simulink model "foc_control"  (R2022b)
settings: Solver=FixedStepAuto  StartTime=0.0  StopTime=0.1  FixedStep=1e-6  RelTol=1e-3
InitFcn:
  | init_pmsm
values from neighbouring files (symbols this model uses):
  B = 0.00001    (= 1e-05)    [init_pmsm.m]
  current_loop_wc = 800    [init_pmsm.m]
  J = 0.0001    [init_pmsm.m]
  Ld = 0.0028    [init_pmsm.m]
  Lq = 0.0028    [init_pmsm.m]
  Pn = 7    [init_pmsm.m]
  Psi = 0.002188    [init_pmsm.m]
  Rs = 5.1    [init_pmsm.m]
  Ts = 1/PWM_Freq    (= 0.000125)    [init_pmsm.m]
  Udc = 12    [init_pmsm.m]
libraries: slpidlib x2, mcbcontrolslib x1, simulink x1
settings Model: Creator=w1545  LastModifiedBy=w1545

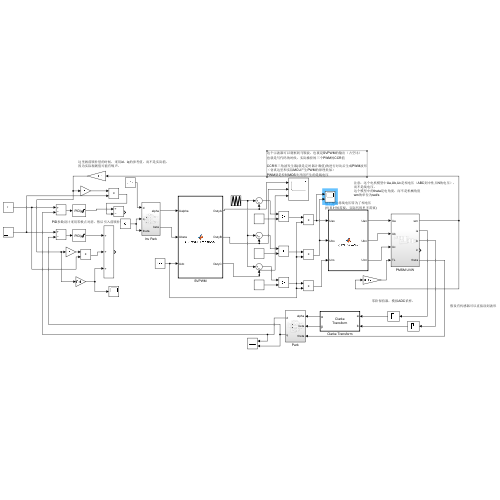
[thumbnail: Simulink's stored preview of the top-level diagram]
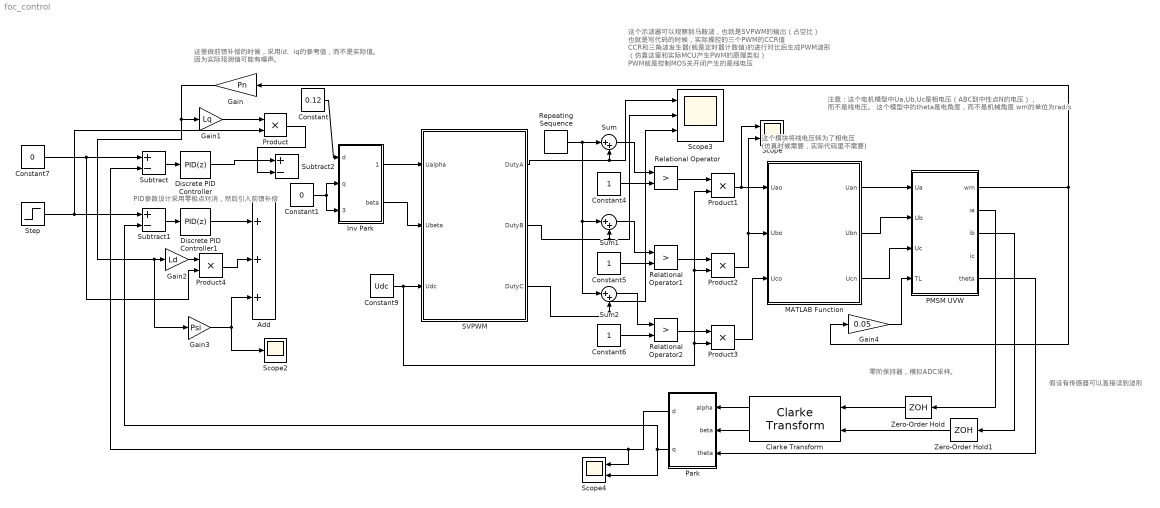
== system foc_control ==
  note: PID参数设计采用零极点对消，然后引入前馈补偿
  note: 假设有传感器可以直接读到波形
  note: 零阶保持器，模拟ADC采样。
  note: 这个模块将线电压转为了相电压
      | (仿真时候需要，实际代码里不需要)
  note: 这个示波器可以观察到马鞍波，也就是SVPWM的输出（占空比）
      | 也就是写代码的时候，实际操控的三个PWM的CCR值
      |
      | CCR和三角波发生器(就是定时器计数值)的进行对比后生成PWM波形
      | （仿真这里和实际MCU产生PWM的原理类似）
      | PWM就是控制MOS关开闭产生的是线电压
  note: 这里做前馈补偿的时候，采用id、iq的参考值，而不是实际值。
      | 因为实际观测值可能有噪声。
  note: 注意：这个电机模型中Ua,Ub,Uc是相电压（ABC到中性点N的电压），
      | 而不是线电压。
      | 这个模型中的theta是电角度，而不是机械角度
      | wm的单位为rad/s
  Add : Sum  Inputs=+++
  Clarke Transform : mcbcontrolslib/Clarke Transform  VariantControl=Variant2
      settings: LibrarySourceBlock=mcbhdllib/Controls/Math Transforms/Clarke Transform
  Constant : Constant  Value=0.12
  Constant1 : Constant  Value=0
  Constant4 : Constant
  Constant5 : Constant
  Constant6 : Constant
  Constant7 : Constant  Value=0
  Constant9 : Constant  Value=Udc
  Discrete PID Controller : slpidlib/PID Controller  Controller=PID  Form=Parallel  TimeDomain=Discrete-time  UseExternalTs=off  SampleTime=Ts  IntegratorMethod=Forward Euler  FilterMethod=Forward Euler  ControllerParametersSource=internal  P=Ld*current_loop_wc  I=Rs*current_loop_wc  UseKiTs=off  D=0  N=100  UseFilter=on  TunerSelectOption=Transfer Function Based (PID Tuner App)  InitialConditionSource=internal  InitialConditionForIntegrator=0  InitialConditionForFilter=0  DifferentiatorICPrevScaledInput=0  ExternalReset=none  TrackingMode=off  Kt=1  LimitOutput=on  SatLimitsSource=internal  UpperSaturationLimit=Udc/sqrt(3)  LowerSaturationLimit=-Udc/sqrt(3)  LinearizeAsGain=off  AntiWindupMode=none  Kb=1  LimitIntegrator=off  UpperIntegratorSaturationLimit=inf  LowerIntegratorSaturationLimit=-inf  POutMin=[]  POutMax=[]  IOutMin=[]  IOutMax=[]  DOutMin=[]  DOutMax=[]  NOutMin=[]  NOutMax=[]  SumOutMin=[]  SumOutMax=[]  SaturationOutMin=[]  SaturationOutMax=[]  PParamMin=[]  PParamMax=[]  IParamMin=[]  IParamMax=[]  DParamMin=[]  DParamMax=[]  NParamMin=[]  NParamMax=[]  KbParamMin=[]  KbParamMax=[]  KtParamMin=[]  KtParamMax=[]  KbOutMin=[]  KbOutMax=[]  KtOutMin=[]  KtOutMax=[]  IntegratorOutMin=[]  IntegratorOutMax=[]  FilterOutMin=[]  FilterOutMax=[]  SumI1OutMin=[]  SumI1OutMax=[]  SumI2OutMin=[]  SumI2OutMax=[]  SumI3OutMin=[]  SumI3OutMax=[]  SumI4OutMin=[]  SumI4OutMax=[]  SumDOutMin=[]  SumDOutMax=[]  DifferentiatorOutMin=[]  DifferentiatorOutMax=[]  FilterDiffOutCoefMin=[]  FilterDiffOutCoefMax=[]  ReciprocalOutMin=[]  ReciprocalOutMax=[]  SumDenOutMin=[]  SumDenOutMax=[]  SumNumOutMin=[]  SumNumOutMax=[]  DivideOutMin=[]  DivideOutMax=[]  UdiffTsProdOutMin=[]  UdiffTsProdOutMax=[]  NTsProdOutMin=[]  NTsProdOutMax=[]  UintegralTsProdOutMin=[]  UintegralTsProdOutMax=[]  UngainTsProdOutMin=[]  UngainTsProdOutMax=[]  ClampingZeroOutDataTypeStr=Inherit: Inherit via back propagation  ClampingZeroOutMin=[]  ClampingZeroOutMax=[]  FilterDenConstantOutDataTypeStr=Inherit: Inherit via back propagation  FilterDenConstantOutMin=[]  FilterDenConstantOutMax=[]  PCopyOutDataTypeStr=Inherit: Inherit via back propagation  PCopyOutMin=[]  PCopyOutMax=[]  NCopyOutDataTypeStr=Inherit: Inherit via back propagation  NCopyOutMin=[]  NCopyOutMax=[]  IntegratorContinuousStateAttributes=''  IntegratorStateMustResolveToSignalObject=off  IntegratorRTWStateStorageClass=Auto  FilterContinuousStateAttributes=''  FilterStateMustResolveToSignalObject=off  FilterRTWStateStorageClass=Auto  ParallelPVariant=InternalParameters  IdealPVariant=Disabled  IVariant=InternalParameters  DVariant=InternalParameters  IntegratorVariant=Discrete  SatVariant=Enabled  AWVariant=Passthrough  PCopyVariant=Disabled  TRVariant=Disabled  FdbkBlocksVariant=Forward  IdealPFdbkVariant=Disabled  SatFdbkVariant=Disabled  DerivativeFilterVariant=ForwardEulerFilter  NVariant=InternalParameters  NCopyVariant=Disabled  FilterICVariant=InternalICsFilter  IntegratorICVariant=InternalICs  ExternalResetVariant=Disabled  TRSumVariant=Passthrough  SumFdbkVariant=Disabled  SumVariant=Sum_PID  TsampFilterVariant=InternalTs  TsampNgainVariant=Passthrough  TsampIntegralVariant=Passthrough  ExternalSaturationOutDataTypeStr=Inherit: Same as second input
      settings: LibrarySourceBlock=hdlsllib/Discrete/Discrete PID Controller
  Discrete PID Controller1 : slpidlib/PID Controller  Controller=PID  Form=Parallel  TimeDomain=Discrete-time  UseExternalTs=off  SampleTime=Ts  IntegratorMethod=Forward Euler  FilterMethod=Forward Euler  ControllerParametersSource=internal  P=Lq*current_loop_wc  I=Rs*current_loop_wc  UseKiTs=off  D=0  N=100  UseFilter=on  TunerSelectOption=Transfer Function Based (PID Tuner App)  InitialConditionSource=internal  InitialConditionForIntegrator=0  InitialConditionForFilter=0  DifferentiatorICPrevScaledInput=0  ExternalReset=none  TrackingMode=off  Kt=1  LimitOutput=on  SatLimitsSource=internal  UpperSaturationLimit=Udc/sqrt(3)  LowerSaturationLimit=-Udc/sqrt(3)  LinearizeAsGain=off  AntiWindupMode=none  Kb=1  LimitIntegrator=off  UpperIntegratorSaturationLimit=inf  LowerIntegratorSaturationLimit=-inf  POutMin=[]  POutMax=[]  IOutMin=[]  IOutMax=[]  DOutMin=[]  DOutMax=[]  NOutMin=[]  NOutMax=[]  SumOutMin=[]  SumOutMax=[]  SaturationOutMin=[]  SaturationOutMax=[]  PParamMin=[]  PParamMax=[]  IParamMin=[]  IParamMax=[]  DParamMin=[]  DParamMax=[]  NParamMin=[]  NParamMax=[]  KbParamMin=[]  KbParamMax=[]  KtParamMin=[]  KtParamMax=[]  KbOutMin=[]  KbOutMax=[]  KtOutMin=[]  KtOutMax=[]  IntegratorOutMin=[]  IntegratorOutMax=[]  FilterOutMin=[]  FilterOutMax=[]  SumI1OutMin=[]  SumI1OutMax=[]  SumI2OutMin=[]  SumI2OutMax=[]  SumI3OutMin=[]  SumI3OutMax=[]  SumI4OutMin=[]  SumI4OutMax=[]  SumDOutMin=[]  SumDOutMax=[]  DifferentiatorOutMin=[]  DifferentiatorOutMax=[]  FilterDiffOutCoefMin=[]  FilterDiffOutCoefMax=[]  ReciprocalOutMin=[]  ReciprocalOutMax=[]  SumDenOutMin=[]  SumDenOutMax=[]  SumNumOutMin=[]  SumNumOutMax=[]  DivideOutMin=[]  DivideOutMax=[]  UdiffTsProdOutMin=[]  UdiffTsProdOutMax=[]  NTsProdOutMin=[]  NTsProdOutMax=[]  UintegralTsProdOutMin=[]  UintegralTsProdOutMax=[]  UngainTsProdOutMin=[]  UngainTsProdOutMax=[]  ClampingZeroOutDataTypeStr=Inherit: Inherit via back propagation  ClampingZeroOutMin=[]  ClampingZeroOutMax=[]  FilterDenConstantOutDataTypeStr=Inherit: Inherit via back propagation  FilterDenConstantOutMin=[]  FilterDenConstantOutMax=[]  PCopyOutDataTypeStr=Inherit: Inherit via back propagation  PCopyOutMin=[]  PCopyOutMax=[]  NCopyOutDataTypeStr=Inherit: Inherit via back propagation  NCopyOutMin=[]  NCopyOutMax=[]  IntegratorContinuousStateAttributes=''  IntegratorStateMustResolveToSignalObject=off  IntegratorRTWStateStorageClass=Auto  FilterContinuousStateAttributes=''  FilterStateMustResolveToSignalObject=off  FilterRTWStateStorageClass=Auto  ParallelPVariant=InternalParameters  IdealPVariant=Disabled  IVariant=InternalParameters  DVariant=InternalParameters  IntegratorVariant=Discrete  SatVariant=Enabled  AWVariant=Passthrough  PCopyVariant=Disabled  TRVariant=Disabled  FdbkBlocksVariant=Forward  IdealPFdbkVariant=Disabled  SatFdbkVariant=Disabled  DerivativeFilterVariant=ForwardEulerFilter  NVariant=InternalParameters  NCopyVariant=Disabled  FilterICVariant=InternalICsFilter  IntegratorICVariant=InternalICs  ExternalResetVariant=Disabled  TRSumVariant=Passthrough  SumFdbkVariant=Disabled  SumVariant=Sum_PID  TsampFilterVariant=InternalTs  TsampNgainVariant=Passthrough  TsampIntegralVariant=Passthrough  ExternalSaturationOutDataTypeStr=Inherit: Same as second input
      settings: LibrarySourceBlock=hdlsllib/Discrete/Discrete PID Controller
  Gain : Gain  Gain=Pn
  Gain1 : Gain  Gain=Lq
  Gain2 : Gain  Gain=Ld
  Gain3 : Gain  Gain=Psi
  Gain4 : Gain  Gain=0.05
  Inv Park : Subsystem
  MATLAB Function : MATLAB Function  TreatAsAtomicUnit=on
  PMSM UVW : Subsystem
  Park : Subsystem
  Product{,1..4} (5 alike) : Product
  Relational Operator : RelationalOperator  Operator=>  OutDataTypeStr=boolean  RndMeth=Simplest  InputSameDT=off
  Relational Operator1 : RelationalOperator  Operator=>  OutDataTypeStr=boolean  RndMeth=Simplest  InputSameDT=off
  Relational Operator2 : RelationalOperator  Operator=>  OutDataTypeStr=boolean  RndMeth=Simplest  InputSameDT=off
  Repeating Sequence : simulink/Sources/Repeating Sequence  rep_seq_t=[0 Ts/2 Ts]  rep_seq_y=[0 1 0]
  SVPWM : MATLAB Function  TreatAsAtomicUnit=on
  Scope : Scope  NumInputPorts=2
  Scope2 : Scope
  Scope3 : Scope  NumInputPorts=3
  Scope4 : Scope  NumInputPorts=2
  Step : Step  Time=0.5  Before=1  After=2  SampleTime=0
  Subtract : Sum  Inputs=+-
  Subtract1 : Sum  Inputs=+-
  Subtract2 : Sum  Inputs=+-
  Sum : Sum  Inputs=|++
  Sum1 : Sum  Inputs=|++
  Sum2 : Sum  Inputs=|++
  Zero-Order Hold : ZeroOrderHold  SampleTime=Ts
  Zero-Order Hold1 : ZeroOrderHold  SampleTime=Ts
  wires:
  MATLAB Function/1(Uan) -> PMSM UVW/1(Ua)
  MATLAB Function/2(Ubn) -> PMSM UVW/2(Ub)
  MATLAB Function/3(Ucn) -> PMSM UVW/3(Uc)
  Gain4/1 -> PMSM UVW/4(TL)
  PMSM UVW/5(theta) -> Park/3(theta)
  Constant4/1 -> Relational Operator/2
  SVPWM/1(DutyA) -> Scope3/1, Sum/2
  Sum/1 -> Relational Operator/1
  Sum1/1 -> Relational Operator1/1
  SVPWM/2(DutyB) -> Scope3/2, Sum1/2
  Constant5/1 -> Relational Operator1/2
  Sum2/1 -> Relational Operator2/1
  SVPWM/3(DutyC) -> Scope3/3, Sum2/2
  Repeating Sequence/1 -> Sum2/1, Sum1/1, Sum/1
  Constant6/1 -> Relational Operator2/2
  Constant9/1 -> SVPWM/3(Udc), Product3/2, Product2/2, Product1/2
  Relational Operator/1 -> Product1/1
  Relational Operator1/1 -> Product2/1
  Relational Operator2/1 -> Product3/1
  Product1/1 -> Scope/1, MATLAB Function/1(Uao)
  Product2/1 -> Scope/2, MATLAB Function/2(Ubo)
  Product3/1 -> MATLAB Function/3(Uco)
  Clarke Transform/1 -> Park/1(alpha)
  Clarke Transform/2 -> Park/2(beta)
  Inv Park/1(alpha) -> SVPWM/1(Ualpha)
  Inv Park/2(beta) -> SVPWM/2(Ubeta)
  Park/1(d) -> Subtract/2, Scope4/1
  Park/2(q) -> Scope4/2, Subtract1/2
  Constant7/1 -> Subtract/1, Product4/2
  Step/1 -> Subtract1/1, Product/2
  Subtract/1 -> Discrete PID Controller/1
  Subtract1/1 -> Discrete PID Controller1/1
  Discrete PID Controller/1 -> Subtract2/1
  PMSM UVW/1(wm) -> Gain4/1, Gain/1
  Gain1/1 -> Product/1
  Product/1 -> Subtract2/2
  Discrete PID Controller1/1 -> Add/1
  Gain2/1 -> Product4/1
  Product4/1 -> Add/2
  Gain3/1 -> Scope2/1, Add/3
  Gain/1 -> Gain3/1, Gain2/1, Gain1/1
  Zero-Order Hold/1 -> Clarke Transform/1
  PMSM UVW/2(ia) -> Zero-Order Hold/1
  Zero-Order Hold1/1 -> Clarke Transform/2
  PMSM UVW/3(ib) -> Zero-Order Hold1/1
  Constant/1 -> Inv Park/1(d)
  Constant1/1 -> Inv Park/3(theta), Inv Park/2(q)

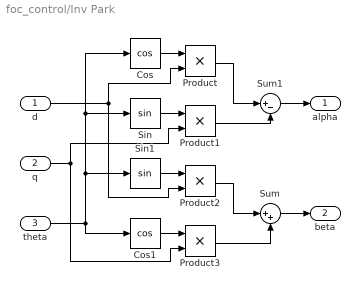
== system foc_control/Inv Park ==
  d : Inport
  q : Inport  Port=2
  theta : Inport  Port=3
  Cos : Trigonometry  Operator=cos
  Cos1 : Trigonometry  Operator=cos
  Product{,1..3} (4 alike) : Product
  Sin : Trigonometry
  Sin1 : Trigonometry
  Sum : Sum  Inputs=|++
  Sum1 : Sum  Inputs=|+-
  alpha : Outport
  beta : Outport  Port=2
  wires:
  theta/1 -> Cos1/1, Cos/1, Sin/1, Sin1/1
  Sum1/1 -> alpha/1
  q/1 -> Product1/2, Product3/2
  d/1 -> Product2/2, Product/2
  Product2/1 -> Sum/1
  Sin1/1 -> Product2/1
  Product3/1 -> Sum/2
  Product1/1 -> Sum1/2
  Sum/1 -> beta/1
  Sin/1 -> Product1/1
  Product/1 -> Sum1/1
  Cos/1 -> Product/1
  Cos1/1 -> Product3/1

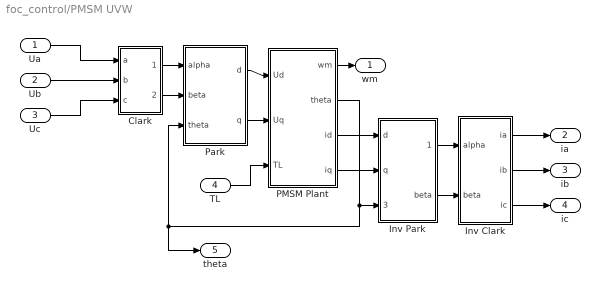
== system foc_control/PMSM UVW ==
  Ua : Inport
  Ub : Inport  Port=2
  Uc : Inport  Port=3
  TL : Inport  Port=4
  Clark : Subsystem
  Inv Clark : Subsystem
  Inv Park : Subsystem
  PMSM Plant : Subsystem
  Park : Subsystem
  wm : Outport
  ia : Outport  Port=2
  ib : Outport  Port=3
  ic : Outport  Port=4
  theta : Outport  Port=5
  wires:
  PMSM Plant/3(id) -> Inv Park/1(d)
  Clark/1(alpha) -> Park/1(alpha)
  Ua/1 -> Clark/1(a)
  Clark/2(beta) -> Park/2(beta)
  Ub/1 -> Clark/2(b)
  Uc/1 -> Clark/3(c)
  Park/1(d) -> PMSM Plant/1(Ud)
  PMSM Plant/2(theta) -> theta/1, Park/3(theta), Inv Park/3(theta)
  Inv Clark/2(ib) -> ib/1
  PMSM Plant/4(iq) -> Inv Park/2(q)
  Park/2(q) -> PMSM Plant/2(Uq)
  Inv Clark/3(ic) -> ic/1
  Inv Park/2(beta) -> Inv Clark/2(beta)
  Inv Park/1(alpha) -> Inv Clark/1(alpha)
  Inv Clark/1(ia) -> ia/1
  TL/1 -> PMSM Plant/3(TL)
  PMSM Plant/1(wm) -> wm/1

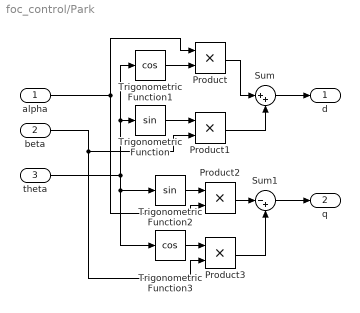
== system foc_control/Park ==
  alpha : Inport
  beta : Inport  Port=2
  theta : Inport  Port=3
  Product{,1..3} (4 alike) : Product
  Sum : Sum  Inputs=|++
  Sum1 : Sum  Inputs=|-+
  Trigonometric Function : Trigonometry
  Trigonometric Function1 : Trigonometry  Operator=cos
  Trigonometric Function2 : Trigonometry
  Trigonometric Function3 : Trigonometry  Operator=cos
  d : Outport
  q : Outport  Port=2
  wires:
  theta/1 -> Trigonometric Function2/1, Trigonometric Function3/1, Trigonometric Function/1, Trigonometric Function1/1
  alpha/1 -> Product2/2, Product/1
  Trigonometric Function1/1 -> Product/2
  Trigonometric Function2/1 -> Product2/1
  Trigonometric Function3/1 -> Product3/1
  Product2/1 -> Sum1/1
  Trigonometric Function/1 -> Product1/1
  Sum/1 -> d/1
  Product3/1 -> Sum1/2
  beta/1 -> Product1/2, Product3/2
  Product1/1 -> Sum/2
  Product/1 -> Sum/1
  Sum1/1 -> q/1

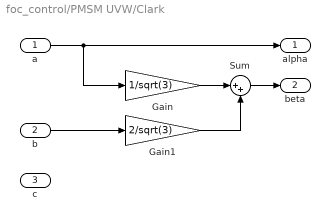
== system foc_control/PMSM UVW/Clark ==
  a : Inport
  b : Inport  Port=2
  c : Inport  Port=3
  Gain : Gain  Gain=1/sqrt(3)
  Gain1 : Gain  Gain=2/sqrt(3)
  Sum : Sum  Inputs=|++
  alpha : Outport
  beta : Outport  Port=2
  wires:
  Sum/1 -> beta/1
  Gain/1 -> Sum/1
  a/1 -> alpha/1, Gain/1
  b/1 -> Gain1/1
  Gain1/1 -> Sum/2

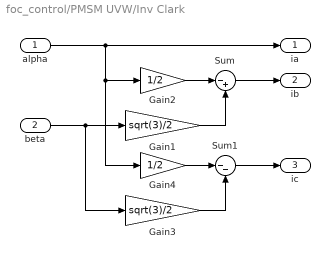
== system foc_control/PMSM UVW/Inv Clark ==
  alpha : Inport
  beta : Inport  Port=2
  Gain1 : Gain  Gain=sqrt(3)/2
  Gain2 : Gain  Gain=1/2
  Gain3 : Gain  Gain=sqrt(3)/2
  Gain4 : Gain  Gain=1/2
  Sum : Sum  Inputs=|-+
  Sum1 : Sum  Inputs=|--
  ia : Outport
  ib : Outport  Port=2
  ic : Outport  Port=3
  wires:
  alpha/1 -> Gain2/1, Gain4/1, ia/1
  Sum/1 -> ib/1
  Sum1/1 -> ic/1
  Gain2/1 -> Sum/1
  beta/1 -> Gain3/1, Gain1/1
  Gain1/1 -> Sum/2
  Gain3/1 -> Sum1/2
  Gain4/1 -> Sum1/1

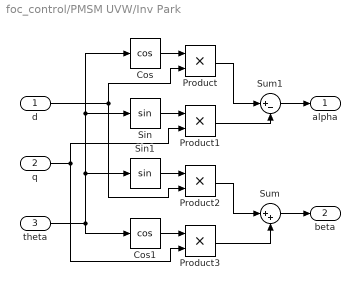
== system foc_control/PMSM UVW/Inv Park ==
  d : Inport
  q : Inport  Port=2
  theta : Inport  Port=3
  Cos : Trigonometry  Operator=cos
  Cos1 : Trigonometry  Operator=cos
  Product{,1..3} (4 alike) : Product
  Sin : Trigonometry
  Sin1 : Trigonometry
  Sum : Sum  Inputs=|++
  Sum1 : Sum  Inputs=|+-
  alpha : Outport
  beta : Outport  Port=2
  wires:
  theta/1 -> Cos1/1, Cos/1, Sin/1, Sin1/1
  Sum1/1 -> alpha/1
  q/1 -> Product1/2, Product3/2
  d/1 -> Product2/2, Product/2
  Product2/1 -> Sum/1
  Sin1/1 -> Product2/1
  Product3/1 -> Sum/2
  Product1/1 -> Sum1/2
  Sum/1 -> beta/1
  Sin/1 -> Product1/1
  Product/1 -> Sum1/1
  Cos/1 -> Product/1
  Cos1/1 -> Product3/1

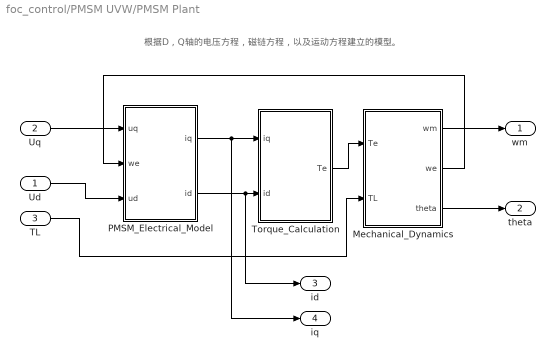
== system foc_control/PMSM UVW/PMSM Plant ==
  note: 根据D，Q轴的电压方程，磁链方程，以及运动方程建立的模型。
  Ud : Inport
  Uq : Inport  Port=2
  TL : Inport  Port=3
  Mechanical_Dynamics : Subsystem
  PMSM_Electrical_Model : Subsystem
  Torque_Calculation : Subsystem
  wm : Outport
  theta : Outport  Port=2
  id : Outport  Port=3
  iq : Outport  Port=4
  wires:
  PMSM_Electrical_Model/2(id) -> id/1, Torque_Calculation/2(id)
  Mechanical_Dynamics/2(we) -> PMSM_Electrical_Model/2(we)
  Mechanical_Dynamics/3(theta) -> theta/1
  Mechanical_Dynamics/1(wm) -> wm/1
  TL/1 -> Mechanical_Dynamics/2(TL)
  PMSM_Electrical_Model/1(iq) -> iq/1, Torque_Calculation/1(iq)
  Uq/1 -> PMSM_Electrical_Model/1(uq)
  Torque_Calculation/1(Te) -> Mechanical_Dynamics/1(Te)
  Ud/1 -> PMSM_Electrical_Model/3(ud)

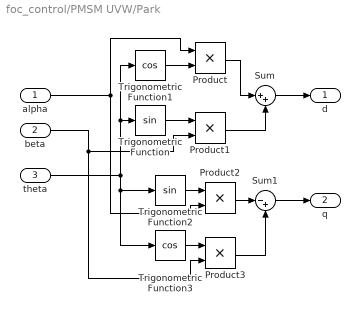
== system foc_control/PMSM UVW/Park ==
  alpha : Inport
  beta : Inport  Port=2
  theta : Inport  Port=3
  Product{,1..3} (4 alike) : Product
  Sum : Sum  Inputs=|++
  Sum1 : Sum  Inputs=|-+
  Trigonometric Function : Trigonometry
  Trigonometric Function1 : Trigonometry  Operator=cos
  Trigonometric Function2 : Trigonometry
  Trigonometric Function3 : Trigonometry  Operator=cos
  d : Outport
  q : Outport  Port=2
  wires:
  theta/1 -> Trigonometric Function2/1, Trigonometric Function3/1, Trigonometric Function/1, Trigonometric Function1/1
  alpha/1 -> Product2/2, Product/1
  Trigonometric Function1/1 -> Product/2
  Trigonometric Function2/1 -> Product2/1
  Trigonometric Function3/1 -> Product3/1
  Product2/1 -> Sum1/1
  Trigonometric Function/1 -> Product1/1
  Sum/1 -> d/1
  Product3/1 -> Sum1/2
  beta/1 -> Product1/2, Product3/2
  Product1/1 -> Sum/2
  Product/1 -> Sum/1
  Sum1/1 -> q/1

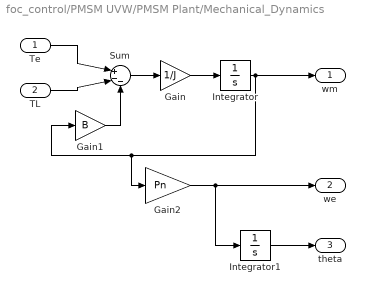
== system foc_control/PMSM UVW/PMSM Plant/Mechanical_Dynamics ==
  Te : Inport
  TL : Inport  Port=2
  Gain : Gain  Gain=1/J
  Gain1 : Gain  Gain=B
  Gain2 : Gain  Gain=Pn
  Integrator : Integrator
  Integrator1 : Integrator
  Sum : Sum  Inputs=|+--
  wm : Outport
  we : Outport  Port=2
  theta : Outport  Port=3
  wires:
  Gain/1 -> Integrator/1
  Gain1/1 -> Sum/3
  Te/1 -> Sum/1
  TL/1 -> Sum/2
  Integrator/1 -> wm/1, Gain2/1, Gain1/1
  Integrator1/1 -> theta/1
  Gain2/1 -> we/1, Integrator1/1
  Sum/1 -> Gain/1

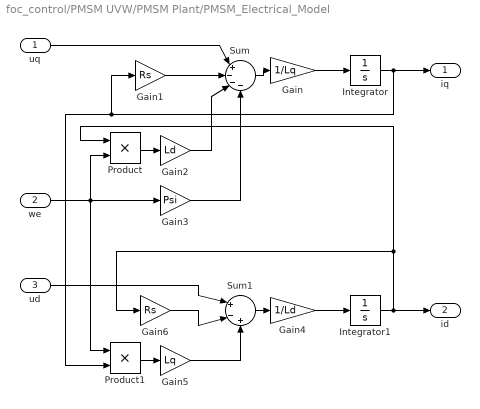
== system foc_control/PMSM UVW/PMSM Plant/PMSM_Electrical_Model ==
  uq : Inport
  we : Inport  Port=2
  ud : Inport  Port=3
  Gain : Gain  Gain=1/Lq
  Gain1 : Gain  Gain=Rs
  Gain2 : Gain  Gain=Ld
  Gain3 : Gain  Gain=Psi
  Gain4 : Gain  Gain=1/Ld
  Gain5 : Gain  Gain=Lq
  Gain6 : Gain  Gain=Rs
  Integrator : Integrator
  Integrator1 : Integrator
  Product : Product
  Product1 : Product
  Sum : Sum  Inputs=|+---
  Sum1 : Sum  Inputs=|+-+
  iq : Outport
  id : Outport  Port=2
  wires:
  Product/1 -> Gain2/1
  Gain/1 -> Integrator/1
  Gain5/1 -> Sum1/3
  we/1 -> Product1/1, Gain3/1, Product/2
  Sum/1 -> Gain/1
  Integrator/1 -> iq/1, Product1/2, Gain1/1
  Gain2/1 -> Sum/3
  Gain3/1 -> Sum/4
  uq/1 -> Sum/1
  Gain1/1 -> Sum/2
  Integrator1/1 -> id/1, Gain6/1, Product/1
  Sum1/1 -> Gain4/1
  Gain6/1 -> Sum1/2
  Gain4/1 -> Integrator1/1
  Product1/1 -> Gain5/1
  ud/1 -> Sum1/1

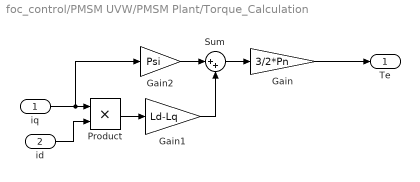
== system foc_control/PMSM UVW/PMSM Plant/Torque_Calculation ==
  iq : Inport
  id : Inport  Port=2
  Gain : Gain  Gain=3/2*Pn
  Gain1 : Gain  Gain=Ld-Lq
  Gain2 : Gain  Gain=Psi
  Product : Product
  Sum : Sum  Inputs=|++
  Te : Outport
  wires:
  id/1 -> Product/2
  Product/1 -> Gain1/1
  Sum/1 -> Gain/1
  Gain1/1 -> Sum/2
  Gain2/1 -> Sum/1
  iq/1 -> Gain2/1, Product/1
  Gain/1 -> Te/1

== matlab function foc_control/MATLAB Function ==
  data: Uao input; Uan output; Ubo input; Uco input; Ubn output; Ucn output
function [Uan, Ubn, Ucn] = Volt2PhaseVolt(Uao, Ubo, Uco)
    % 计算电机中性点电压 (三相桥臂电压的平均值)
    Un = (Uao + Ubo + Uco) / 3.0;
    
    % 计算真实的相电压
    Uan = Uao - Un;
    Ubn = Ubo - Un;
    Ucn = Uco - Un;
end

== matlab function foc_control/SVPWM ==
  data: Ualpha input; DutyA output; Ubeta input; Udc input; DutyB output; DutyC output
function[DutyA, DutyB, DutyC] = SVPWM_Traditional(Ualpha, Ubeta, Udc)
    % 输入说明：
    % Ualpha, Ubeta: 逆Park变换输出的静止坐标系电压参考值
    % Udc: 直流母线电压
    % 输出说明：
    % DutyA, DutyB, DutyC: 输出的三相占空比 (范围 0.0 ~ 1.0)
    
    % --- 1. 定义临时变量判断扇区 ---
    U1 = Ubeta;
    U2 = (sqrt(3)/2) * Ualpha - 0.5 * Ubeta;
    U3 = -(sqrt(3)/2) * Ualpha - 0.5 * Ubeta;
    
    % --- 2. 扇区判断 (Sector 1 ~ 6) ---
    A = 0; B = 0; C = 0;
    if (U1 > 0), A = 1; end
    if (U2 > 0), B = 1; end
    if (U3 > 0), C = 1; end
    
    N = A + 2*B + 4*C; % N 的取值范围是 1~6，但对应关系不是顺序的
    
    % --- 3. 计算基本矢量作用时间 X, Y, Z (这里已归一化，视Ts=1) ---
    K = sqrt(3) / Udc; 
    X = K * Ubeta;
    Y = K * ((sqrt(3)/2) * Ualpha + 0.5 * Ubeta);
    Z = K * (-(sqrt(3)/2) * Ualpha + 0.5 * Ubeta);
    
    % --- 4. 提取当前扇区的两个非零基本矢量时间 T1 和 T2 ---
    T1 = 0; T2 = 0;
    switch N
        case 3  % 第 1 扇区
            T1 = -Z; T2 = X;
        case 1  % 第 2 扇区
            T1 = Z;  T2 = Y;
        case 5  % 第 3 扇区
            T1 = X;  T2 = -Y;
        case 4  % 第 4 扇区
            T1 = -X; T2 = Z;
        case 6  % 第 5 扇区
            T1 = -Y; T2 = -Z;
        case 2  % 第 6 扇区
            T1 = Y;  T2 = -X;
    end
    
    % --- 5. 过调制处理 (如果T1+T2大于整个周期1，则等比例缩小) ---
    if (T1 + T2 > 1.0)
        sumT = T1 + T2;
        T1 = T1 / sumT;
        T2 = T2 / sumT;
    end
    
    % --- 6. 计算七段式中心对齐的发波切换时间 ---
    % Ta, Tb, Tc 代表在半个载波周期内的切换点
    Ta = (1 - T1 - T2) / 4;
    Tb = Ta + T1 / 2;
    Tc = Tb + T2 / 2;
    
    % 将切换时间转换为实际的等效占空比 (0~1)
    Da = 1 - 2*Ta;
    Db = 1 - 2*Tb;
    Dc = 1 - 2*Tc;
    
    % --- 7. 根据扇区将占空比映射到 A, B, C 三相 ---
    DutyA = 0; DutyB = 0; DutyC = 0;
    switch N
        case 3  % 第 1 扇区
            DutyA = Da; DutyB = Db; DutyC = Dc;
        case 1  % 第 2 扇区
            DutyA = Db; DutyB = Da; DutyC = Dc;
        case 5  % 第 3 扇区
            DutyA = Dc; DutyB = Da; DutyC = Db;
        case 4  % 第 4 扇区
            DutyA = Dc; DutyB = Db; DutyC = Da;
        case 6  % 第 5 扇区
            DutyA = Db; DutyB = Dc; DutyC = Da;
        case 2  % 第 6 扇区
            DutyA = Da; DutyB = Dc; DutyC = Db;
    end
end
